simulink model "crazyflie_backup2"  (R2018b)
settings: Solver=FixedStepDiscrete  StartTime=0.0  StopTime=25  FixedStep=0.01  RelTol=1e-3
undefined symbols (not defined in the file or in its folder): DiscIntNeverNeededParam
settings Model: PauseTimes=7  Creator=Zrean  LastModifiedBy=orjan
settings OptimizationCC: DefaultParameterBehavior=Inlined  UseDivisionForNetSlopeComputation=on  UseFloatMulNetSlope=on  UseSpecifiedMinMax=on  InlineInvariantSignals=on  PassReuseOutputArgsAs=Individual arguments  ZeroExternalMemoryAtStartup=off  ZeroInternalMemoryAtStartup=off  NoFixptDivByZeroProtection=on  EfficientFloat2IntCast=on  LifeSpan=1
settings DebuggingCC: AlgebraicLoopMsg=error  ParameterTunabilityLossMsg=error
settings HardwareCC: ProdBitPerPointer=32  ProdBitPerSizeT=32  ProdBitPerPtrDiffT=32  ProdLargestAtomicInteger=Long  ProdLargestAtomicFloat=Double  ProdWordSize=32  ProdHWDeviceType=ARM Compatible->ARM Cortex
settings SFSimCC: SimUseLocalCustomCode=off  MATLABDynamicMemAlloc=off
settings RTWCC: SystemTargetFile=ert.tlc  GenCodeOnly=on  TemplateMakefile=ert_default_tmf  GenerateReport=on  RTWUseLocalCustomCode=off  BuildConfiguration=Faster Runs  IncludeHyperlinkInReport=on  LaunchReport=on  GenerateTraceInfo=on  GenerateTraceReport=on  GenerateTraceReportSl=on  GenerateTraceReportSf=on  GenerateTraceReportEml=on  GenerateCodeMetricsReport=on
settings CodeAppCC: ForceParamTrailComments=on  IgnoreCustomStorageClasses=off  OperatorAnnotations=on  SimulinkDataObjDesc=on  SFDataObjDesc=on  MATLABFcnDesc=on  CustomSymbolStrGlobalVar=rt$N$M  CustomSymbolStrType=$N$M  CustomSymbolStrFcn=$N$M$F  CustomSymbolStrMacro=$N$M  InsertBlockDesc=on  StateflowObjectComments=on  MATLABSourceComments=on
settings ERTTargetCC: TargetLangStandard=C99 (ISO)  MultiwordLength=2048  CombineSignalStateStructs=on  SuppressErrorStatus=on  SupportAbsoluteTime=off  SupportNonFinite=off  SupportComplex=off  InlinedParameterPlacement=NonHierarchical  ERTCustomFileTemplate=crazyflie_wrapper.tlc  ERTFilePackagingFormat=CompactWithDataFile
settings SimscapeCC: SimscapeNormalizeSystem=off

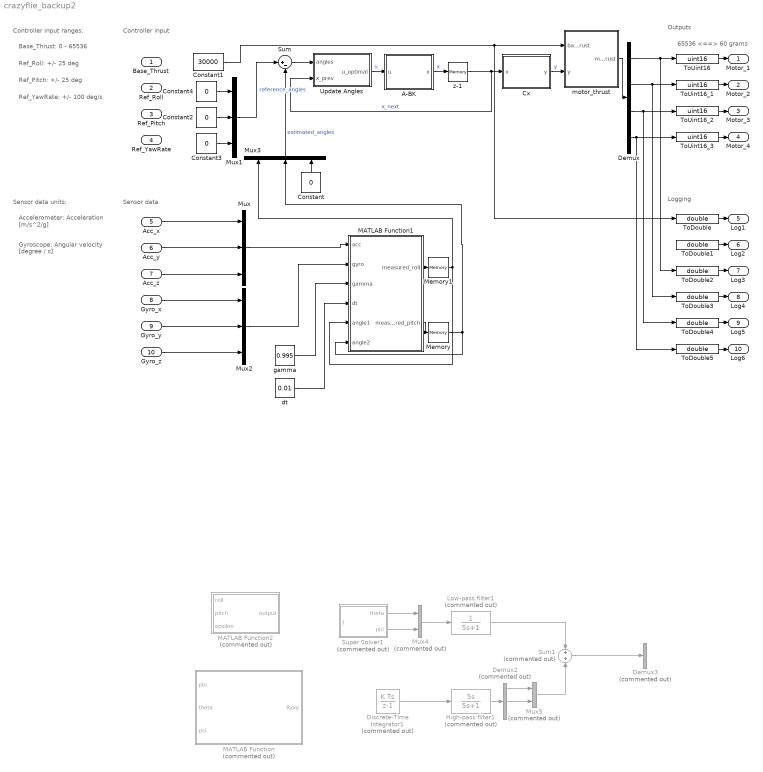
== system crazyflie_backup2 ==
  note: 65536 <==> 60 grams
  note: Logging
  note: Outputs
  note: Sensor data
  note: Controller input
  note: Ref_Roll: +/- 25 deg
  note: Base_Thrust: 0 - 65536
  note: Ref_Pitch: +/- 25 deg
  note: Ref_YawRate: +/- 100 deg/s
  note: Controller input ranges:
  note: Gyroscope:
      | Angular velocity [degree / s]
  note: Accelerometer:
      | Acceleration [m/s^2/g]
  note: Sensor data units:
  Base_Thrust : Inport  OutDataTypeStr=double
  Ref_Roll : Inport  Port=2  OutDataTypeStr=double
  Ref_Pitch : Inport  Port=3  OutDataTypeStr=double
  Ref_YawRate : Inport  Port=4  OutDataTypeStr=double
  Acc_x : Inport  Port=5  OutDataTypeStr=double  PortDimensions=1
  Acc_y : Inport  Port=6  OutDataTypeStr=double  PortDimensions=1
  Acc_z : Inport  Port=7  OutDataTypeStr=double  PortDimensions=1
  Gyro_x : Inport  Port=8  OutDataTypeStr=double  PortDimensions=1
  Gyro_y : Inport  Port=9  OutDataTypeStr=double  PortDimensions=1
  Gyro_z : Inport  Port=10  OutDataTypeStr=double  PortDimensions=1
  A-BK : MATLAB Function  TreatAsAtomicUnit=on
  Constant{,2..4} (4 alike) : Constant  Value=0
  Constant1 : Constant  Value=30000
  Cx : MATLAB Function  TreatAsAtomicUnit=on
  Demux : Demux
  Demux2 : Demux  Commented=on  Outputs=3
  Demux3 : Demux  Commented=on  Outputs=2
  Discrete-Time Integrator1 : DiscreteIntegrator  Commented=on  SampleTime=-1  ICPrevOutput=DiscIntNeverNeededParam  ICPrevScaledInput=DiscIntNeverNeededParam
  High-pass filter1 : TransferFcn  Commented=on  Numerator=[5 0]  Denominator=[5 1]
  Low-pass filter1 : TransferFcn  Commented=on  Denominator=[5 1]
  MATLAB Function : MATLAB Function  Commented=on  TreatAsAtomicUnit=on
  MATLAB Function1 : MATLAB Function  TreatAsAtomicUnit=on
  MATLAB Function2 : MATLAB Function  Commented=on  TreatAsAtomicUnit=on
  Memory : Memory  InheritSampleTime=on
  Memory1 : Memory  InheritSampleTime=on
  Mux{,1..3} (4 alike) : Mux  Inputs=3
  Mux4 : Mux  Commented=on  Inputs=2
  Mux5 : Mux  Commented=on  Inputs=2
  Sum : Sum  Inputs=|+-
  Sum1 : Sum  Commented=on  Inputs=+|+
  Super Solver1 : MATLAB Function  Commented=on  TreatAsAtomicUnit=on
  ToDouble{,1..5} (6 alike) : DataTypeConversion  OutDataTypeStr=double  SaturateOnIntegerOverflow=on
  ToUint16 : DataTypeConversion  OutDataTypeStr=uint16  SaturateOnIntegerOverflow=on
  ToUint16_1 : DataTypeConversion  OutDataTypeStr=uint16  SaturateOnIntegerOverflow=on
  ToUint16_2 : DataTypeConversion  OutDataTypeStr=uint16  SaturateOnIntegerOverflow=on
  ToUint16_3 : DataTypeConversion  OutDataTypeStr=uint16  SaturateOnIntegerOverflow=on
  Update Angles : MATLAB Function  TreatAsAtomicUnit=on
  dt : Constant  Value=0.01
  gamma : Constant  Value=0.995
  motor_thrust : MATLAB Function  TreatAsAtomicUnit=on
  z-1 : Memory  InitialCondition=[0;0;0;0;0;0;0;0;0;0;0;0]  InheritSampleTime=on
  Motor_1 : Outport  OutDataTypeStr=uint16  LockScale=on
  Motor_2 : Outport  Port=2  OutDataTypeStr=uint16  LockScale=on
  Motor_3 : Outport  Port=3  OutDataTypeStr=uint16  LockScale=on
  Motor_4 : Outport  Port=4  OutDataTypeStr=uint16  LockScale=on
  Log1 : Outport  Port=5  OutDataTypeStr=double
  Log2 : Outport  Port=6  OutDataTypeStr=double
  Log3 : Outport  Port=7  OutDataTypeStr=double
  Log4 : Outport  Port=8  OutDataTypeStr=double
  Log5 : Outport  Port=9  OutDataTypeStr=double
  Log6 : Outport  Port=10  OutDataTypeStr=double
  wires:
  ToUint16/1 -> Motor_1/1
  ToUint16_1/1 -> Motor_2/1
  ToUint16_2/1 -> Motor_3/1
  ToUint16_3/1 -> Motor_4/1
  ToDouble/1 -> Log1/1
  ToDouble1/1 -> Log2/1
  ToDouble2/1 -> Log3/1
  ToDouble3/1 -> Log4/1
  ToDouble4/1 -> Log5/1
  ToDouble5/1 -> Log6/1
  Acc_z/1 -> Mux/3
  Acc_y/1 -> Mux/2
  Acc_x/1 -> Mux/1
  Gyro_y/1 -> Mux2/2
  Gyro_x/1 -> Mux2/1
  Gyro_z/1 -> Mux2/3
  Mux4/1 -> Low-pass filter1/1
  Discrete-Time Integrator1/1 -> High-pass filter1/1
  Sum1/1 -> Demux3/1
  Mux5/1 -> Sum1/2
  Low-pass filter1/1 -> Sum1/1
  High-pass filter1/1 -> Demux2/1
  Super Solver1/1(theta) -> Mux4/1
  Demux2/1 -> Mux5/1
  Demux2/2 -> Mux5/2
  Super Solver1/2(phi) -> Mux4/2
  Mux/1 -> MATLAB Function1/1(acc)
  Mux2/1 -> MATLAB Function1/2(gyro)
  gamma/1 -> MATLAB Function1/3(gamma)
  dt/1 -> MATLAB Function1/4(dt)
  MATLAB Function1/2(measured_pitch) -> Memory/1
  MATLAB Function1/1(measured_roll) -> Memory1/1
  Memory1/1 -> Mux3/1, MATLAB Function1/5(angle1)
  Memory/1 -> MATLAB Function1/6(angle2), Mux3/2
  Mux1/1 -> Sum/1  "reference_angles"
  Mux3/1 -> Sum/2  "estimated_angles"
  Constant/1 -> Mux3/3
  Sum/1 -> Update Angles/1(angles)
  Constant1/1 -> ToDouble/1, motor_thrust/1(base_thrust)
  Cx/1(y) -> motor_thrust/2(y)  "y"
  Update Angles/1(u_optimal) -> A-BK/1(u)  "u"
  A-BK/1(x) -> z-1/1  "x"
  z-1/1 -> Update Angles/2(x_prev), Cx/1(x)  "x_next"
  Constant4/1 -> Mux1/1
  Constant2/1 -> Mux1/2
  Constant3/1 -> Mux1/3
  Demux/4 -> ToDouble5/1, ToUint16_3/1
  Demux/3 -> ToDouble4/1, ToUint16_2/1
  Demux/2 -> ToDouble3/1, ToUint16_1/1
  Demux/1 -> ToDouble2/1, ToUint16/1
  motor_thrust/1(motor_thrust) -> Demux/1

== matlab function crazyflie_backup2/MATLAB Function1 ==
  data: acc input; measured_roll output; gyro input; gamma input; dt input; angle1 input; angle2 input; measured_pitch output
function [measured_roll, measured_pitch] = fcn(acc,gyro,gamma,dt,angle1, angle2)
	if nargin < 5
		angle1 = 0;
		angle2 = 0;
	end
	measured_roll = (gamma)*(angle1+gyro(1)*dt)+(1-gamma)*acc(1);
	measured_pitch = (gamma)*(angle2+gyro(2)*dt)+(1-gamma)*acc(2);
end

== matlab function crazyflie_backup2/MATLAB Function ==
  data: phi input; Rzxy output; theta input; psi input
% gives the rotation matrix with Tait Bryan Angles ZYX
function Rzxy = Tati_Bryan_Euler_Angles_ZYX(phi, theta, psi)
s1=sin(phi);
s2=sin(theta);
s3=sin(psi);
c1=cos(phi);
c2=cos(theta);
c3=cos(psi);
Rzxy = [c1*c2,	c1*s2*s3-c3*s1,		s1*s3+c1*c3*s2;
			c2*s1,	c1*c3+s1*s2*s3,		c3*s1*s2-c1*s3
			-s2,		c2*s3,							c2*c3];
end

== matlab function crazyflie_backup2/Super Solver1 ==
  data: f input; theta output; phi output
function [theta, phi] = fcn(f)
	f_hat = f./norm(f);
	theta = atan2(f_hat(2), f_hat(3));
	phi = atan2(-f_hat(1), sqrt(f_hat(2)^2 + f_hat(3)^2));
end

== matlab function crazyflie_backup2/MATLAB Function2 ==
  data: roll input; output output; pitch input; epsilon input
function output  = fcn(roll, pitch, epsilon)
	roll_output = [0 0 0 0];
	pitch_output = [0 0 0 0];
	if roll < -epsilon
		roll_output = [0 0 1 1];
	elseif roll > epsilon
		roll_output = [1 1 0 0];
	end
	if pitch < -epsilon
		pitch_output = [0 1 1 0];
	elseif pitch > epsilon
		pitch_output = [1 0 0 1];
	end
	output = roll_output+pitch_output;
	output=output/max(max(output),1);
end

== matlab function crazyflie_backup2/A-BK ==
  data: x output; u input
function x = fcn(u)
%function output = fcn(input,A,B)

% AB=load('linAB.mat'); %Loading Linearized system
% A=AB.A;
% B=AB.B;
% subs(A,base_thrust,basethrust);
% subs(B,base_thrust,basethrust);
% 
% Q=eye(A);
% R=eye(length(B(1,:)));
% 
% [K,L]=dare(A,B,Q,R);

%x=[input;zeros(9,1)];%extending inputs

%output=(A-B*K)*input;

 ABK = [0,0,0,1,0,0,0,0,0,0,0,0;0,0,0,0,1,0,0,0,0,0,0,0;0,0,0,0,0,1,0,0,0,0,0,0;0,0,0,0,0,0,0,4444444.44444444,0,0,0,0;0,0,0,0,0,0,-4444444.44444444,0,0,0,0,0;0,0,-74.0740740740740,0,0,-75.0674136898265,0,0,0,0,0,0;0,0,0,0,0,0,0,0,0,1,0,0;0,0,0,0,0,0,0,0,0,0,1,0;0,0,0,0,0,0,0,0,0,0,0,1;0,4663.35654976073,0,0,4667.33956996207,0,-17709871.8680313,0,0,-7560.86225547451,0,0;-4530.21057584702,0,0,-4534.10062792606,0,0,0,-17296543.3593679,0,0,-7424.00798627341,0;0,0,0,0,0,0,0,0,-3346860.22674978,0,0,-3346861.22674963];
 
x=(ABK)*u;

== matlab function crazyflie_backup2/Update Angles ==
  data: angles input; u_optimal output; x_prev input
function u_optimal = fcn(angles,x_prev)

u_optimal = [x_prev(1:6);angles;x_prev(10:12)];

== matlab function crazyflie_backup2/Cx ==
  data: x input; y output
function y = fcn(x)

C=zeros(4,12);
C(:,7:8)=[ 1  1
           1 -1
          -1 -1
          -1  1];

y = C*x;

== matlab function crazyflie_backup2/motor_thrust ==
  data: base_thrust input; motor_thrust output; y input
function motor_thrust = fcn(base_thrust,y)
    motor_thrust = y+base_thrust;
    
    for i = 1:length(motor_thrust)
        motor_thrust(i) = max([0,motor_thrust(i)]);
        motor_thrust(i) = min([65536,motor_thrust(i)]);
    end
end
